simulink model "fmcw_controller_test"  (R2025b)
settings: Solver=FixedStepDiscrete  StartTime=0.0  StopTime=2.298e-05  FixedStep=5e-09  RelTol=1e-3
settings Model: DataTypeOverride=Off  Creator=kimsteph  LastModifiedBy=kimsteph
settings OptimizationCC: BlockReduction=off  ConditionallyExecuteInputs=off  DefaultParameterBehavior=Inlined  InheritOutputTypeSmallerThanSingle=on
settings DebuggingCC: ArtificialAlgebraicLoopMsg=error  SingleTaskRateTransMsg=error
settings HardwareCC: ProdBitPerPointer=32.0  ProdBitPerSizeT=32.0  ProdBitPerPtrDiffT=32.0  ProdLargestAtomicFloat=None  ProdIntDivRoundTo=Undefined  ProdEndianess=Unspecified  ProdWordSize=32.0  ProdHWDeviceType=ASIC/FPGA->ASIC/FPGA  TargetBitPerPointer=64.0  TargetBitPerSizeT=64.0  TargetBitPerPtrDiffT=64.0  TargetLongLongMode=on  TargetIntDivRoundTo=Zero  TargetEndianess=LittleEndian  TargetWordSize=64.0  TargetHWDeviceType=Custom Processor->MATLAB Host Computer  ProdEqTarget=off

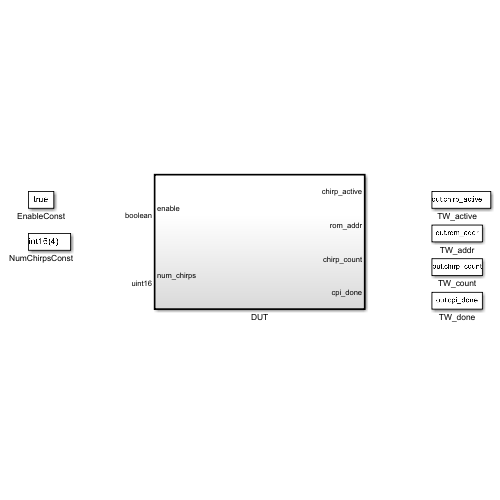
[thumbnail: Simulink's stored preview of the top-level diagram]
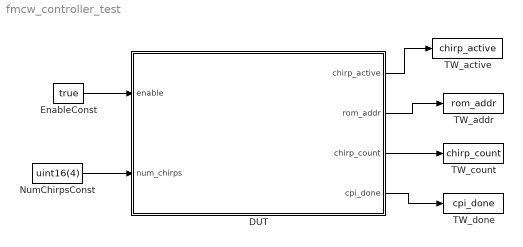
== system fmcw_controller_test ==
  DUT : Subsystem  TreatAsAtomicUnit=on
  EnableConst : Constant  Value=true  OutDataTypeStr=boolean
  NumChirpsConst : Constant  Value=uint16(4)  OutDataTypeStr=uint16
  TW_active : ToWorkspace  VariableName=chirp_active  SaveFormat=Timeseries  SampleTime=-1
  TW_addr : ToWorkspace  VariableName=rom_addr  SaveFormat=Timeseries  SampleTime=-1
  TW_count : ToWorkspace  VariableName=chirp_count  SaveFormat=Timeseries  SampleTime=-1
  TW_done : ToWorkspace  VariableName=cpi_done  SaveFormat=Timeseries  SampleTime=-1
  wires:
  EnableConst/1 -> DUT/1(enable)
  NumChirpsConst/1 -> DUT/2(num_chirps)
  DUT/2(rom_addr) -> TW_addr/1
  DUT/1(chirp_active) -> TW_active/1
  DUT/3(chirp_count) -> TW_count/1
  DUT/4(cpi_done) -> TW_done/1

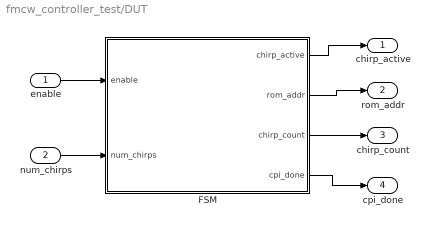
== system fmcw_controller_test/DUT ==
  enable : Inport  OutDataTypeStr=boolean
  num_chirps : Inport  Port=2  OutDataTypeStr=uint16
  FSM : Stateflow chart  TreatAsAtomicUnit=on
  chirp_active : Outport
  rom_addr : Outport  Port=2
  chirp_count : Outport  Port=3
  cpi_done : Outport  Port=4
  wires:
  FSM/4(cpi_done) -> cpi_done/1
  enable/1 -> FSM/1(enable)
  num_chirps/1 -> FSM/2(num_chirps)
  FSM/1(chirp_active) -> chirp_active/1
  FSM/2(rom_addr) -> rom_addr/1
  FSM/3(chirp_count) -> chirp_count/1

== stateflow chart fmcw_controller_test/DUT/FSM ==
  state IDLE
    entry: chirp_active=false; rom_addr=uint16(0); chirp_count=uint16(0);
    cpi_done=false; sample_cnt=uint16(0);
  state CHIRP_ACTIVE
    entry: chirp_active=true; sample_cnt=uint16(0);
    during: rom_addr=sample_cnt; sample_cnt=sample_cnt+uint16(1);
  state CPI_DONE
    entry: cpi_done=true; chirp_active=false;
    during: sample_cnt=sample_cnt+uint16(1);
  state FLYBACK
    entry: chirp_active=false; chirp_count=chirp_count+uint16(1); sample_cnt=uint16(0);
    during: sample_cnt=sample_cnt+uint16(1);
  (default) -> IDLE
  CPI_DONE -> IDLE : [sample_cnt >= uint16(100)]
  IDLE -> CHIRP_ACTIVE : [enable]
  FLYBACK -> CHIRP_ACTIVE [order 1] : [sample_cnt >= uint16(50) && chirp_count < num_chirps]
  FLYBACK -> CPI_DONE [order 2] : [chirp_count >= num_chirps]
  CHIRP_ACTIVE -> FLYBACK : [sample_cnt >= uint16(1024)]
  data: enable input boolean; num_chirps input uint16; chirp_active output boolean; rom_addr output uint16; chirp_count output uint16; cpi_done output boolean; sample_cnt local uint16
